simulink model "Resp18e_updatedPulse"  (Simulink 7.3)
settings: Solver=ode23  StartTime=0.0  StopTime=20  FixedStep=0.01  MaxStep=0.05  RelTol=1e-6
values from neighbouring files (symbols this model uses):
  alpha_CO2_brain = 2.9/1e3*760/P_stp/K_stp    (= 0.00097047576489)    [initialize_parameters.m]
  alpha_CO2_fat = 0.9/K_stp/P_stp    (= 0.000396292281489)    [initialize_parameters.m]
  alpha_CO2_heart = 2.4/1e3*760/P_stp/K_stp    (= 0.00080315235715)    [initialize_parameters.m]
  alpha_CO2_lean = 4.2/1e3*760/P_stp/K_stp    (= 0.00140551662501)    [initialize_parameters.m]
  alpha_CO2_lungtiss_fast = alpha_CO2_lungtiss_fast./0.1333    [initialize_parameters.m]
  alpha_CO2_muscle = 4.2/1e3*760/P_stp/K_stp    (= 0.00140551662501)    [initialize_parameters.m]
  alpha_CO2_other = 3.0/1e3*760/P_stp/K_stp    (= 0.00100394044644)    [initialize_parameters.m]
  alpha_O2_fat = 5*0.024/K_stp/P_stp    (= 5.28389708651e-05)    [initialize_parameters.m]
  alpha_O2_tissue = 0.024/K_stp/P_stp    (= 1.0567794173e-05)    [initialize_parameters.m]
  BOHRF0 = O2_SHIFT - T_BLOOD_M_37 * (0.024 + BOHRF * 0.0147) - BOHRF1 * 7.4    (= -3.552)    [initialize_parameters.m]
  BOHRF1 = BOHRF * (1 - T_BLOOD_M_37 * 0.0065)    (= 0.48)    [initialize_parameters.m]
  C_a_CO2_i = 20.8e-3    (= 0.0208)    [initialize_parameters.m]    (also in resp18e_ic_norm.mat = 0.0202734801806)
  C_a_O2_i = 8.95e-3    (= 0.00895)    [initialize_parameters.m]    (also in resp18e_ic_norm.mat = 0.00918087581167)
  CAP_O2 = 0.01 * CAP_O2    (= 0.201)    [initialize_parameters.m]
  Cardiac_duty_cycle = 40    [initialize_parameters.m]
  Co_CO2_brain = 401*K_Co_CO2/1e3/K_stp    (= 0.0107345869894)    [initialize_parameters.m]
  Co_CO2_heart = 487*K_Co_CO2/1e3/K_stp    (= 0.0130367677403)    [initialize_parameters.m]
  Co_CO2_lean = 342*K_Co_CO2/1e3/K_stp    (= 0.00915518391618)    [initialize_parameters.m]
  Co_CO2_muscle = 342*K_Co_CO2/1e3/K_stp    (= 0.00915518391618)    [initialize_parameters.m]
  Co_CO2_other = 355*K_Co_CO2/1e3/K_stp    (= 0.00950318798317)    [initialize_parameters.m]
  DH2ODS = DH2ODS + 0.007 * HB_MEQ * (HB_MEQ - 9) / (13.5 * (13.5 - 9))    (= 0.00498709726946)    [initialize_parameters.m]
  F_insp_alv_alvds = F_v_alv_deadspace / F_insp_hivq    (= 0.00299401197605)    [initialize_parameters.m]
  F_insp_alv_hivq = F_v_alv_hivq      / F_insp_hivq    (= 0.997005988024)    [initialize_parameters.m]
  F_insp_alv_lovq = F_v_alv_lovq      / F_insp_lovq    (= 0.5)    [initialize_parameters.m]
  F_insp_alv_midvq = F_v_alv_midvq     / F_insp_lovq    (= 0.5)    [initialize_parameters.m]
  F_insp_hivq = F_v_alv_deadspace + F_v_alv_hivq    (= 0.334)    [initialize_parameters.m]
  F_insp_lovq = F_v_alv_midvq     + F_v_alv_lovq    (= 0.666)    [initialize_parameters.m]
  Fi_CO2_param_est = 0.01    [initialize_parameters.m]
  Fi_error = 1e-6    (= 1e-06)    [initialize_parameters.m]
  Fi_N2_mean = 1-(Fi_O2_mean + Fi_N2O_mean)    (= 0.65)    [initialize_parameters.m]
  Fi_O2_mean = 0.35    [initialize_parameters.m]
  Fi_O2_param_est = 0.01    [initialize_parameters.m]
  Fq_brain = 0.114    [initialize_parameters.m]
  Fq_error = 1e-8    (= 1e-08)    [initialize_parameters.m]
  Fq_fat = 0.103    [initialize_parameters.m]
  Fq_heart = 0.041    [initialize_parameters.m]
  Fq_hepatic = 0.069    [initialize_parameters.m]
  Fq_kidneys = 0.215    [initialize_parameters.m]
  Fq_lean = 0.090    (= 0.09)    [initialize_parameters.m]
  Fq_lungs_anatomicalshunt = 0.01    [initialize_parameters.m]
  Fq_lungs_hivq = (1-Fq_lungs_pulmshunt-Fq_lungs_anatomicalshunt)    *F_v_alv_hivq/(F_v_alv_hivq+F_v_alv_midvq+F_v_alv_lovq)    (= 0.3)    [initialize_parameters.m]
  Fq_lungs_lovq = (1-Fq_lungs_pulmshunt-Fq_lungs_anatomicalshunt)    *F_v_alv_lovq/(F_v_alv_hivq+F_v_alv_midvq+F_v_alv_lovq)    (= 0.3)    [initialize_parameters.m]
  Fq_lungs_midvq = (1-Fq_lungs_pulmshunt-Fq_lungs_anatomicalshunt)    *F_v_alv_midvq/(F_v_alv_hivq+F_v_alv_midvq+F_v_alv_lovq)    (= 0.3)    [initialize_parameters.m]
  Fq_lungs_pulmshunt = 0.09    [initialize_parameters.m]
  Fq_muscle = 0.096    [initialize_parameters.m]
  Fq_pershunt = 0.101    [initialize_parameters.m]
  Fq_portal = 0.171    [initialize_parameters.m]
  FRC = 2.2    [initialize_parameters.m]
  H2OB = H2OVC + 0.938 * (1 - VC_74)    (= 0.840191964286)    [initialize_parameters.m]
  k_CO2_lungtiss_fast_alvds = k_CO2_lungtiss_fast*F_v_alv_deadspace    (= 3.63090772693e-07)    [initialize_parameters.m]
  k_CO2_lungtiss_fast_hivq = k_CO2_lungtiss_fast*F_v_alv_hivq    (= 0.000120909227307)    [initialize_parameters.m]
  k_CO2_lungtiss_fast_lovq = k_CO2_lungtiss_fast*F_v_alv_lovq    (= 0.000120909227307)    [initialize_parameters.m]
  k_CO2_lungtiss_fast_midvq = k_CO2_lungtiss_fast*F_v_alv_midvq    (= 0.000120909227307)    [initialize_parameters.m]
  k_CO2_lungtiss_slow_alvds = k_CO2_lungtiss_slow*F_v_alv_deadspace    (= 4.95123780945e-09)    [initialize_parameters.m]
  k_CO2_lungtiss_slow_hivq = k_CO2_lungtiss_slow*F_v_alv_hivq    (= 1.64876219055e-06)    [initialize_parameters.m]
  k_CO2_lungtiss_slow_lovq = k_CO2_lungtiss_slow*F_v_alv_lovq    (= 1.64876219055e-06)    [initialize_parameters.m]
  k_CO2_lungtiss_slow_midvq = k_CO2_lungtiss_slow*F_v_alv_midvq    (= 1.64876219055e-06)    [initialize_parameters.m]
  K_diff_CO2_hivq = K_diff_CO2*F_v_alv_hivq    (= 0.0014985)    [initialize_parameters.m]
  K_diff_CO2_lovq = K_diff_CO2*F_v_alv_lovq    (= 0.0014985)    [initialize_parameters.m]
  K_diff_CO2_midvq = K_diff_CO2*F_v_alv_midvq    (= 0.0014985)    [initialize_parameters.m]
  K_diff_O2_hivq = K_diff_O2*F_v_alv_hivq    (= 7.326e-05)    [initialize_parameters.m]
  K_diff_O2_lovq = K_diff_O2*F_v_alv_lovq    (= 7.326e-05)    [initialize_parameters.m]
  K_diff_O2_midvq = K_diff_O2*F_v_alv_midvq    (= 7.326e-05)    [initialize_parameters.m]
  K_exp_alv_alvds = 1/1    (= 1)    [initialize_parameters.m]
  K_exp_alv_hivq = 1/1    (= 1)    [initialize_parameters.m]
  K_press = 760/101.325    (= 7.50061682704)    [initialize_parameters.m]
  K_stp = R*(T_stp+273.15)/(P_stp*1000)    (= 22.4135311621)    [initialize_parameters.m]
  Kg_alv = R*(T_alv+273.15)/(P_baro*1000)    (= 25.3668469802)    [initialize_parameters.m]
  LN10 = 2.30258509299405    (= 2.30258509299)    [initialize_parameters.m]
  m_alv_alvds_i = (FRC-V_deadspace_total)/Kg_alv * F_v_alv_deadspace    [initialize_parameters.m]
  m_alv_hivq_i = (FRC-V_deadspace_total)/Kg_alv * F_v_alv_hivq    [initialize_parameters.m]
  m_alv_lovq_i = (FRC-V_deadspace_total)/Kg_alv * F_v_alv_lovq    [initialize_parameters.m]
  m_alv_midvq_i = (FRC-V_deadspace_total)/Kg_alv * F_v_alv_midvq    [initialize_parameters.m]
  m_CO2_alv_alvds_i = F_CO2_i * m_alv_alvds_i    [initialize_parameters.m]
  m_CO2_alv_hivq_i = F_CO2_i * m_alv_hivq_i    [initialize_parameters.m]
  m_CO2_alv_lovq_i = F_CO2_i * m_alv_lovq_i    [initialize_parameters.m]
  m_CO2_alv_midvq_i = F_CO2_i * m_alv_midvq_i    [initialize_parameters.m]
  m_CO2_brain_b_i = C_a_CO2_i*Vb_brain    (= 0.002184)    [initialize_parameters.m]
  m_CO2_brain_t_i = (Co_CO2_brain  + alpha_CO2_brain *P_v_CO2_i)* Vt_brain    (= 0.0171268217946)    [initialize_parameters.m]
  m_CO2_common_b_i = C_a_CO2_i*Vb_common    (= 0.0170421333333)    [initialize_parameters.m]
  m_CO2_ds0_i = F_CO2_i*m_ds0_i    (= 0.000985538329597)    [initialize_parameters.m]
  m_CO2_ds_large_i = F_CO2_i * m_deadspace_large_1    [initialize_parameters.m]
  m_CO2_ds_med_hivq1_i = F_CO2_i * m_deadspace_med_hivq_1    [initialize_parameters.m]
  m_CO2_ds_med_hivq2_i = F_CO2_i * m_deadspace_med_hivq_2    [initialize_parameters.m]
  m_CO2_ds_med_lovq1_i = F_CO2_i * m_deadspace_med_lovq_1    [initialize_parameters.m]
  m_CO2_ds_med_lovq2_i = F_CO2_i * m_deadspace_med_lovq_2    [initialize_parameters.m]
  m_CO2_ds_small_alvds_i = F_CO2_i * m_deadspace_small_alvdeadspace    [initialize_parameters.m]
  m_CO2_ds_small_hivq_i = F_CO2_i * m_deadspace_small_hivq    [initialize_parameters.m]
  m_CO2_ds_small_lovq_i = F_CO2_i * m_deadspace_small_lovq    [initialize_parameters.m]
  m_CO2_ds_small_midvq_i = F_CO2_i * m_deadspace_small_midvq    [initialize_parameters.m]
  m_CO2_fat_b_i = C_a_CO2_i*Vb_fat    (= 0.0116896)    [initialize_parameters.m]
  m_CO2_fat_t_i = P_a_CO2_i*alpha_CO2_fat*Vt_fat    (= 0.0302752719501)    [initialize_parameters.m]
  m_CO2_heart_b_i = C_a_CO2_i*Vb_heart    (= 0.000832)    [initialize_parameters.m]
  m_CO2_heart_t_i = (Co_CO2_heart  + alpha_CO2_heart *P_v_CO2_i)* Vt_heart    (= 0.00402544335149)    [initialize_parameters.m]
  m_CO2_hepatic_b_i = C_a_CO2_i*Vb_hepatic    (= 0.0019136)    [initialize_parameters.m]
  m_CO2_kidneys_b_i = C_a_CO2_i*Vb_kidneys    (= 0.0012064)    [initialize_parameters.m]
  m_CO2_kidneys_t_i = (Co_CO2_other  + alpha_CO2_other *P_v_CO2_i)* Vt_kidneys    (= 0.0045902552907)    [initialize_parameters.m]
  m_CO2_lean_b_i = C_a_CO2_i*Vb_lean    (= 0.0191984)    [initialize_parameters.m]
  m_CO2_lean_t_i = (Co_CO2_lean   + alpha_CO2_lean  *P_v_CO2_i)* Vt_lean    (= 0.0884995401953)    [initialize_parameters.m]
  m_CO2_liver_t_i = (Co_CO2_other  + alpha_CO2_other *P_v_CO2_i)* Vt_liver    (= 0.0187019339777)    [initialize_parameters.m]
  m_CO2_lungtiss_fast_alvds_i = F_CO2_i*(P_baro-P_A_H2O)*V_lungtiss_alvds *alpha_CO2_lungtiss_fast(2)    [initialize_parameters.m]
  m_CO2_lungtiss_fast_hivq_i = F_CO2_i*(P_baro-P_A_H2O)*V_lungtiss_hivq  *alpha_CO2_lungtiss_fast(2)    [initialize_parameters.m]
  m_CO2_lungtiss_fast_lovq_i = F_CO2_i*(P_baro-P_A_H2O)*V_lungtiss_lovq  *alpha_CO2_lungtiss_fast(2)    [initialize_parameters.m]
  m_CO2_lungtiss_fast_midvq_i = F_CO2_i*(P_baro-P_A_H2O)*V_lungtiss_midvq *alpha_CO2_lungtiss_fast(2)    [initialize_parameters.m]
  m_CO2_lungtiss_slow_alvds_i = F_CO2_i*(P_baro-P_A_H2O)*V_lungtiss_alvds*alpha_CO2_lungtiss_slow    [initialize_parameters.m]
  m_CO2_lungtiss_slow_hivq_i = F_CO2_i*(P_baro-P_A_H2O)*V_lungtiss_hivq *alpha_CO2_lungtiss_slow    [initialize_parameters.m]
  m_CO2_lungtiss_slow_lovq_i = F_CO2_i*(P_baro-P_A_H2O)*V_lungtiss_lovq *alpha_CO2_lungtiss_slow    [initialize_parameters.m]
  m_CO2_lungtiss_slow_midvq_i = F_CO2_i*(P_baro-P_A_H2O)*V_lungtiss_midvq*alpha_CO2_lungtiss_slow    [initialize_parameters.m]
  m_CO2_LV_b_i = C_a_CO2_i*Vb_LV    (= 0.00391733333333)    [initialize_parameters.m]
  m_CO2_muscle_b_i = C_a_CO2_i*Vb_muscle    (= 0.0201344)    [initialize_parameters.m]
  m_CO2_muscle_t_i = (Co_CO2_muscle + alpha_CO2_muscle*P_v_CO2_i)* Vt_muscle    (= 0.363660431061)    [initialize_parameters.m]
  m_CO2_pershunt_b_i = C_a_CO2_i*Vb_pershunt    (= 0.0027248)    [initialize_parameters.m]
  m_CO2_portal_b_i = C_a_CO2_i*Vb_portal    (= 0.0210912)    [initialize_parameters.m]
  m_CO2_portal_t_i = (Co_CO2_other  + alpha_CO2_other *P_v_CO2_i)* Vt_portal    (= 0.0164739329706)    [initialize_parameters.m]
  m_CO2_pulmcap_b_hivq_i = C_a_CO2_i*Vb_pulmcap_hivq    (= 0.000630933333333)    [initialize_parameters.m]
  m_CO2_pulmcap_b_lovq_i = C_a_CO2_i*Vb_pulmcap_lovq    (= 0.000630933333333)    [initialize_parameters.m]
  m_CO2_pulmcap_b_midvq_i = C_a_CO2_i*Vb_pulmcap_midvq    (= 0.000630933333333)    [initialize_parameters.m]
  m_CO2_pulmcap_b_pulmshunt_i = C_a_CO2_i*Vb_pulmcap_pulmshunt    (= 0.0001872)    [initialize_parameters.m]
  m_CO2_RV_b_i = C_v_CO2_i*Vb_RV    (= 0.004181)    [initialize_parameters.m]
  m_N2_alv_alvds_i = Fi_N2_mean * (m_alv_alvds_i - m_CO2_alv_alvds_i)    [initialize_parameters.m]
  ... (+122 more)
undefined symbols (not defined in the file or in its folder): AH2OVC, AHCO3B, DHCO3BDS, litres, mole
libraries: simulink x28
(part 3 of 8)

== system Resp18e_updatedPulse/Patient/Airways + alveoli/Series dead Space alv dead sp ==
  Insp flow in : Inport  PortDimensions=4  OutDataType=sfix(16)  OutScaling=2^0
  Exp flow in : Inport  Port=2  PortDimensions=4  OutDataType=sfix(16)  OutScaling=2^0
  1/u : Math  Operator=reciprocal  OutDataType=sfix(16)  OutScaling=2^0  SaturateOnIntegerOverflow=on
  CO2 : Integrator  InitialCondition=m_CO2_ds_small_alvds_i
  N2 : Integrator  InitialCondition=m_N2_ds_small_alvds_i
  N2O : Integrator  InitialCondition=m_N2O_ds_small_alvds_i
  N2O O2 CO2 N2 : Demux
  "N2O O2 CO2 N2 " : Demux
  N2O,O2 CO2,N22 : Mux
  N2O,O2 CO2,N23 : Mux
  O2 : Integrator  InitialCondition=m_O2_ds_small_alvds_i
  P{2..13} (12 alike) : Product  OutDataType=sfix(16)  OutScaling=2^0  SaturateOnIntegerOverflow=on  RndMeth=Zero  InputSameDT=on  OutDataTypeStr=Inherit: Same as first input
  Vds gas vol : Sum  Inputs=++++  OutDataType=sfix(16)  OutScaling=2^0  SaturateOnIntegerOverflow=on  InputSameDT=on  OutDataTypeStr=Inherit: Same as first input
  sum : Sum  Inputs=--++  OutDataType=sfix(16)  OutScaling=2^0  SaturateOnIntegerOverflow=on  InputSameDT=on  OutDataTypeStr=Inherit: Same as first input
  sum1 : Sum  Inputs=+-+-  OutDataType=sfix(16)  OutScaling=2^0  SaturateOnIntegerOverflow=on  InputSameDT=on  OutDataTypeStr=Inherit: Same as first input
  sum2 : Sum  Inputs=-++-  OutDataType=sfix(16)  OutScaling=2^0  SaturateOnIntegerOverflow=on  InputSameDT=on  OutDataTypeStr=Inherit: Same as first input
  sum3 : Sum  Inputs=-++-  OutDataType=sfix(16)  OutScaling=2^0  SaturateOnIntegerOverflow=on  InputSameDT=on  OutDataTypeStr=Inherit: Same as first input
  sum4 : Sum  Inputs=++++  OutDataType=sfix(16)  OutScaling=2^0  SaturateOnIntegerOverflow=on  InputSameDT=on  OutDataTypeStr=Inherit: Same as first input
  sum5 : Sum  Inputs=++++  OutDataType=sfix(16)  OutScaling=2^0  SaturateOnIntegerOverflow=on  InputSameDT=on  OutDataTypeStr=Inherit: Same as first input
  Insp flow  Out: : Outport  OutDataType=sfix(16)  OutScaling=2^0
  Exp flow  Out: : Outport  Port=2  OutDataType=sfix(16)  OutScaling=2^0
  wires:
  Insp flow in/1 -> "N2O O2 CO2 N2 "/1
  "N2O O2 CO2 N2 "/4 -> sum4/4, sum3/3
  "N2O O2 CO2 N2 "/3 -> sum4/3, sum2/3
  "N2O O2 CO2 N2 "/2 -> sum4/2, sum1/3
  "N2O O2 CO2 N2 "/1 -> sum4/1, sum/4
  Exp flow in/1 -> N2O O2 CO2 N2/1
  N2O O2 CO2 N2/4 -> sum5/4, sum3/2
  N2O O2 CO2 N2/3 -> sum5/3, sum2/2
  N2O O2 CO2 N2/2 -> sum5/2, sum1/1
  N2O O2 CO2 N2/1 -> sum5/1, sum/3
  sum5/1 -> P6/2, P5/2, P10/2, P11/1
  sum4/1 -> P13/1, P9/1, P7/1, P4/1
  N2/1 -> Vds gas vol/4, P12/2
  P5/1 -> sum/1, N2O,O2 CO2,N23/1
  P6/1 -> sum1/4, N2O,O2 CO2,N23/2
  O2/1 -> Vds gas vol/2, P3/2
  N2O/1 -> Vds gas vol/1, P2/1
  P7/1 -> sum1/2, N2O,O2 CO2,N22/2
  1/u/1 -> P2/2, P3/1, P8/1, P12/1
  Vds gas vol/1 -> 1/u/1
  sum1/1 -> O2/1
  sum/1 -> N2O/1
  sum2/1 -> CO2/1
  P2/1 -> P5/1, P4/2
  CO2/1 -> P8/2, Vds gas vol/3
  P8/1 -> P10/1, P9/2
  P10/1 -> sum2/4, N2O,O2 CO2,N23/3
  N2O,O2 CO2,N23/1 -> Exp flow  Out:/1
  N2O,O2 CO2,N22/1 -> Insp flow  Out:/1
  P4/1 -> N2O,O2 CO2,N22/1, sum/2
  P9/1 -> N2O,O2 CO2,N22/3, sum2/1
  sum3/1 -> N2/1
  P12/1 -> P11/2, P13/2
  P13/1 -> sum3/1, N2O,O2 CO2,N22/4
  P3/1 -> P6/1, P7/2
  P11/1 -> sum3/4, N2O,O2 CO2,N23/4

== system Resp18e_updatedPulse/Patient/Airways + alveoli/Series dead Space hi V/Q ==
  Insp flow in : Inport  PortDimensions=4  OutDataType=sfix(16)  OutScaling=2^0
  Exp flow in : Inport  Port=2  PortDimensions=4  OutDataType=sfix(16)  OutScaling=2^0
  1/u : Math  Operator=reciprocal  OutDataType=sfix(16)  OutScaling=2^0  SaturateOnIntegerOverflow=on
  CO2 : Integrator  InitialCondition=m_CO2_ds_small_hivq_i
  N2 : Integrator  InitialCondition=m_N2_ds_small_hivq_i
  N2O : Integrator  InitialCondition=m_N2O_ds_small_hivq_i
  N2O O2 CO2 N2 : Demux
  "N2O O2 CO2 N2 " : Demux
  N2O,O2 CO2,N22 : Mux
  N2O,O2 CO2,N23 : Mux
  O2 : Integrator  InitialCondition=m_O2_ds_small_hivq_i
  P{2..13} (12 alike) : Product  OutDataType=sfix(16)  OutScaling=2^0  SaturateOnIntegerOverflow=on  RndMeth=Zero  InputSameDT=on  OutDataTypeStr=Inherit: Same as first input
  Vds gas vol : Sum  Inputs=++++  OutDataType=sfix(16)  OutScaling=2^0  SaturateOnIntegerOverflow=on  InputSameDT=on  OutDataTypeStr=Inherit: Same as first input
  sum : Sum  Inputs=--++  OutDataType=sfix(16)  OutScaling=2^0  SaturateOnIntegerOverflow=on  InputSameDT=on  OutDataTypeStr=Inherit: Same as first input
  sum1 : Sum  Inputs=+-+-  OutDataType=sfix(16)  OutScaling=2^0  SaturateOnIntegerOverflow=on  InputSameDT=on  OutDataTypeStr=Inherit: Same as first input
  sum2 : Sum  Inputs=-++-  OutDataType=sfix(16)  OutScaling=2^0  SaturateOnIntegerOverflow=on  InputSameDT=on  OutDataTypeStr=Inherit: Same as first input
  sum3 : Sum  Inputs=-++-  OutDataType=sfix(16)  OutScaling=2^0  SaturateOnIntegerOverflow=on  InputSameDT=on  OutDataTypeStr=Inherit: Same as first input
  sum4 : Sum  Inputs=++++  OutDataType=sfix(16)  OutScaling=2^0  SaturateOnIntegerOverflow=on  InputSameDT=on  OutDataTypeStr=Inherit: Same as first input
  sum5 : Sum  Inputs=++++  OutDataType=sfix(16)  OutScaling=2^0  SaturateOnIntegerOverflow=on  InputSameDT=on  OutDataTypeStr=Inherit: Same as first input
  Insp flow  Out: : Outport  OutDataType=sfix(16)  OutScaling=2^0
  Exp flow  Out: : Outport  Port=2  OutDataType=sfix(16)  OutScaling=2^0
  wires:
  P11/1 -> N2O,O2 CO2,N23/4, sum3/4
  P3/1 -> P7/2, P6/1
  P13/1 -> N2O,O2 CO2,N22/4, sum3/1
  P12/1 -> P13/2, P11/2
  sum3/1 -> N2/1
  P9/1 -> sum2/1, N2O,O2 CO2,N22/3
  P4/1 -> sum/2, N2O,O2 CO2,N22/1
  N2O,O2 CO2,N22/1 -> Insp flow  Out:/1
  N2O,O2 CO2,N23/1 -> Exp flow  Out:/1
  P10/1 -> N2O,O2 CO2,N23/3, sum2/4
  P8/1 -> P9/2, P10/1
  CO2/1 -> Vds gas vol/3, P8/2
  P2/1 -> P4/2, P5/1
  sum2/1 -> CO2/1
  sum/1 -> N2O/1
  sum1/1 -> O2/1
  Vds gas vol/1 -> 1/u/1
  1/u/1 -> P12/1, P8/1, P3/1, P2/2
  P7/1 -> N2O,O2 CO2,N22/2, sum1/2
  N2O/1 -> P2/1, Vds gas vol/1
  O2/1 -> P3/2, Vds gas vol/2
  P6/1 -> N2O,O2 CO2,N23/2, sum1/4
  P5/1 -> N2O,O2 CO2,N23/1, sum/1
  N2/1 -> P12/2, Vds gas vol/4
  sum4/1 -> P4/1, P7/1, P9/1, P13/1
  sum5/1 -> P11/1, P10/2, P5/2, P6/2
  N2O O2 CO2 N2/1 -> sum/3, sum5/1
  N2O O2 CO2 N2/2 -> sum1/1, sum5/2
  N2O O2 CO2 N2/3 -> sum2/2, sum5/3
  N2O O2 CO2 N2/4 -> sum3/2, sum5/4
  Exp flow in/1 -> N2O O2 CO2 N2/1
  "N2O O2 CO2 N2 "/1 -> sum/4, sum4/1
  "N2O O2 CO2 N2 "/2 -> sum1/3, sum4/2
  "N2O O2 CO2 N2 "/3 -> sum2/3, sum4/3
  "N2O O2 CO2 N2 "/4 -> sum3/3, sum4/4
  Insp flow in/1 -> "N2O O2 CO2 N2 "/1

== system Resp18e_updatedPulse/Patient/Airways + alveoli/Series dead Space lo V/Q ==
  Insp flow in : Inport  PortDimensions=4  OutDataType=sfix(16)  OutScaling=2^0
  Exp flow in : Inport  Port=2  PortDimensions=4  OutDataType=sfix(16)  OutScaling=2^0
  1/u : Math  Operator=reciprocal  OutDataType=sfix(16)  OutScaling=2^0  SaturateOnIntegerOverflow=on
  CO2 : Integrator  InitialCondition=m_CO2_ds_small_lovq_i
  N2 : Integrator  InitialCondition=m_N2_ds_small_lovq_i
  N2O : Integrator  InitialCondition=m_N2O_ds_small_lovq_i
  N2O O2 CO2 N2 : Demux
  "N2O O2 CO2 N2 " : Demux
  N2O,O2 CO2,N22 : Mux
  N2O,O2 CO2,N23 : Mux
  O2 : Integrator  InitialCondition=m_O2_ds_small_lovq_i
  P{2..13} (12 alike) : Product  OutDataType=sfix(16)  OutScaling=2^0  SaturateOnIntegerOverflow=on  RndMeth=Zero  InputSameDT=on  OutDataTypeStr=Inherit: Same as first input
  Vds gas vol : Sum  Inputs=++++  OutDataType=sfix(16)  OutScaling=2^0  SaturateOnIntegerOverflow=on  InputSameDT=on  OutDataTypeStr=Inherit: Same as first input
  sum : Sum  Inputs=--++  OutDataType=sfix(16)  OutScaling=2^0  SaturateOnIntegerOverflow=on  InputSameDT=on  OutDataTypeStr=Inherit: Same as first input
  sum1 : Sum  Inputs=+-+-  OutDataType=sfix(16)  OutScaling=2^0  SaturateOnIntegerOverflow=on  InputSameDT=on  OutDataTypeStr=Inherit: Same as first input
  sum2 : Sum  Inputs=-++-  OutDataType=sfix(16)  OutScaling=2^0  SaturateOnIntegerOverflow=on  InputSameDT=on  OutDataTypeStr=Inherit: Same as first input
  sum3 : Sum  Inputs=-++-  OutDataType=sfix(16)  OutScaling=2^0  SaturateOnIntegerOverflow=on  InputSameDT=on  OutDataTypeStr=Inherit: Same as first input
  sum4 : Sum  Inputs=++++  OutDataType=sfix(16)  OutScaling=2^0  SaturateOnIntegerOverflow=on  InputSameDT=on  OutDataTypeStr=Inherit: Same as first input
  sum5 : Sum  Inputs=++++  OutDataType=sfix(16)  OutScaling=2^0  SaturateOnIntegerOverflow=on  InputSameDT=on  OutDataTypeStr=Inherit: Same as first input
  Insp flow  Out: : Outport  OutDataType=sfix(16)  OutScaling=2^0
  Exp flow  Out: : Outport  Port=2  OutDataType=sfix(16)  OutScaling=2^0
  wires:
  P11/1 -> N2O,O2 CO2,N23/4, sum3/4
  P3/1 -> P7/2, P6/1
  P13/1 -> N2O,O2 CO2,N22/4, sum3/1
  P12/1 -> P13/2, P11/2
  sum3/1 -> N2/1
  P9/1 -> sum2/1, N2O,O2 CO2,N22/3
  P4/1 -> sum/2, N2O,O2 CO2,N22/1
  N2O,O2 CO2,N22/1 -> Insp flow  Out:/1
  N2O,O2 CO2,N23/1 -> Exp flow  Out:/1
  P10/1 -> N2O,O2 CO2,N23/3, sum2/4
  P8/1 -> P9/2, P10/1
  CO2/1 -> Vds gas vol/3, P8/2
  P2/1 -> P4/2, P5/1
  sum2/1 -> CO2/1
  sum/1 -> N2O/1
  sum1/1 -> O2/1
  Vds gas vol/1 -> 1/u/1
  1/u/1 -> P12/1, P8/1, P3/1, P2/2
  P7/1 -> N2O,O2 CO2,N22/2, sum1/2
  N2O/1 -> P2/1, Vds gas vol/1
  O2/1 -> P3/2, Vds gas vol/2
  P6/1 -> N2O,O2 CO2,N23/2, sum1/4
  P5/1 -> N2O,O2 CO2,N23/1, sum/1
  N2/1 -> P12/2, Vds gas vol/4
  sum4/1 -> P4/1, P7/1, P9/1, P13/1
  sum5/1 -> P11/1, P10/2, P5/2, P6/2
  N2O O2 CO2 N2/1 -> sum/3, sum5/1
  N2O O2 CO2 N2/2 -> sum1/1, sum5/2
  N2O O2 CO2 N2/3 -> sum2/2, sum5/3
  N2O O2 CO2 N2/4 -> sum3/2, sum5/4
  Exp flow in/1 -> N2O O2 CO2 N2/1
  "N2O O2 CO2 N2 "/1 -> sum/4, sum4/1
  "N2O O2 CO2 N2 "/2 -> sum1/3, sum4/2
  "N2O O2 CO2 N2 "/3 -> sum2/3, sum4/3
  "N2O O2 CO2 N2 "/4 -> sum3/3, sum4/4
  Insp flow in/1 -> "N2O O2 CO2 N2 "/1

== system Resp18e_updatedPulse/Patient/Airways + alveoli/Series dead Space mid V/Q ==
  Insp flow in : Inport  PortDimensions=4  OutDataType=sfix(16)  OutScaling=2^0
  Exp flow in : Inport  Port=2  PortDimensions=4  OutDataType=sfix(16)  OutScaling=2^0
  1/u : Math  Operator=reciprocal  OutDataType=sfix(16)  OutScaling=2^0  SaturateOnIntegerOverflow=on
  CO2 : Integrator  InitialCondition=m_CO2_ds_small_midvq_i
  N2 : Integrator  InitialCondition=m_N2_ds_small_midvq_i
  N2O : Integrator  InitialCondition=m_N2O_ds_small_midvq_i
  N2O O2 CO2 N2 : Demux
  "N2O O2 CO2 N2 " : Demux
  N2O,O2 CO2,N22 : Mux
  N2O,O2 CO2,N23 : Mux
  O2 : Integrator  InitialCondition=m_O2_ds_small_midvq_i
  P{2..13} (12 alike) : Product  OutDataType=sfix(16)  OutScaling=2^0  SaturateOnIntegerOverflow=on  RndMeth=Zero  InputSameDT=on  OutDataTypeStr=Inherit: Same as first input
  Sum Exp flow : Sum  Inputs=++++  OutDataType=sfix(16)  OutScaling=2^0  SaturateOnIntegerOverflow=on  InputSameDT=on  OutDataTypeStr=Inherit: Same as first input
  Sum Insp flow : Sum  Inputs=++++  OutDataType=sfix(16)  OutScaling=2^0  SaturateOnIntegerOverflow=on  InputSameDT=on  OutDataTypeStr=Inherit: Same as first input
  Vds gas vol : Sum  Inputs=++++  OutDataType=sfix(16)  OutScaling=2^0  SaturateOnIntegerOverflow=on  InputSameDT=on  OutDataTypeStr=Inherit: Same as first input
  sum : Sum  Inputs=--++  OutDataType=sfix(16)  OutScaling=2^0  SaturateOnIntegerOverflow=on  InputSameDT=on  OutDataTypeStr=Inherit: Same as first input
  sum1 : Sum  Inputs=+-+-  OutDataType=sfix(16)  OutScaling=2^0  SaturateOnIntegerOverflow=on  InputSameDT=on  OutDataTypeStr=Inherit: Same as first input
  sum2 : Sum  Inputs=-++-  OutDataType=sfix(16)  OutScaling=2^0  SaturateOnIntegerOverflow=on  InputSameDT=on  OutDataTypeStr=Inherit: Same as first input
  sum3 : Sum  Inputs=-++-  OutDataType=sfix(16)  OutScaling=2^0  SaturateOnIntegerOverflow=on  InputSameDT=on  OutDataTypeStr=Inherit: Same as first input
  Insp flow  Out: : Outport  OutDataType=sfix(16)  OutScaling=2^0
  Exp flow  Out: : Outport  Port=2  OutDataType=sfix(16)  OutScaling=2^0
  wires:
  Insp flow in/1 -> "N2O O2 CO2 N2 "/1
  "N2O O2 CO2 N2 "/4 -> Sum Insp flow/4, sum3/3
  "N2O O2 CO2 N2 "/3 -> Sum Insp flow/3, sum2/3
  "N2O O2 CO2 N2 "/2 -> Sum Insp flow/2, sum1/3
  "N2O O2 CO2 N2 "/1 -> Sum Insp flow/1, sum/4
  Exp flow in/1 -> N2O O2 CO2 N2/1
  N2O O2 CO2 N2/4 -> Sum Exp flow/4, sum3/2
  N2O O2 CO2 N2/3 -> Sum Exp flow/3, sum2/2
  N2O O2 CO2 N2/2 -> Sum Exp flow/2, sum1/1
  N2O O2 CO2 N2/1 -> Sum Exp flow/1, sum/3
  Sum Exp flow/1 -> P6/2, P5/2, P10/2, P11/1
  Sum Insp flow/1 -> P13/1, P9/1, P7/1, P4/1
  N2/1 -> Vds gas vol/4, P12/2
  P5/1 -> sum/1, N2O,O2 CO2,N23/1
  P6/1 -> sum1/4, N2O,O2 CO2,N23/2
  O2/1 -> Vds gas vol/2, P3/2
  N2O/1 -> Vds gas vol/1, P2/1
  P7/1 -> sum1/2, N2O,O2 CO2,N22/2
  1/u/1 -> P2/2, P3/1, P8/1, P12/1
  Vds gas vol/1 -> 1/u/1
  sum1/1 -> O2/1
  sum/1 -> N2O/1
  sum2/1 -> CO2/1
  P2/1 -> P5/1, P4/2
  CO2/1 -> P8/2, Vds gas vol/3
  P8/1 -> P10/1, P9/2
  P10/1 -> sum2/4, N2O,O2 CO2,N23/3
  N2O,O2 CO2,N23/1 -> Exp flow  Out:/1
  N2O,O2 CO2,N22/1 -> Insp flow  Out:/1
  P4/1 -> N2O,O2 CO2,N22/1, sum/2
  P9/1 -> N2O,O2 CO2,N22/3, sum2/1
  sum3/1 -> N2/1
  P12/1 -> P11/2, P13/2
  P13/1 -> sum3/1, N2O,O2 CO2,N22/4
  P3/1 -> P6/1, P7/2
  P11/1 -> sum3/4, N2O,O2 CO2,N23/4

== system Resp18e_updatedPulse/Patient/Airways + alveoli/Series deadspace large_1 ==
  mdot insp total : Inport  PortDimensions=1  OutDataType=sfix(16)  OutScaling=2^0
  Insp flow in : Inport  Port=2  PortDimensions=4  OutDataType=sfix(16)  OutScaling=2^0
  mdot exp Total : Inport  Port=3  PortDimensions=1  OutDataType=sfix(16)  OutScaling=2^0
  Exp flow in : Inport  Port=4  PortDimensions=4  OutDataType=sfix(16)  OutScaling=2^0
  1/u : Math  Operator=reciprocal  OutDataType=sfix(16)  OutScaling=2^0  SaturateOnIntegerOverflow=on
  CO2 : Integrator  InitialCondition=m_CO2_ds_large_i
  N2 : Integrator  InitialCondition=m_N2_ds_large_i
  N2O : Integrator  InitialCondition=m_N2O_ds_large_i
  N2O,O2 CO2,N2 : Demux
  N2O,O2 CO2,N21 : Demux
  N2O,O2 CO2,N22 : Mux
  N2O,O2 CO2,N23 : Mux
  O2 : Integrator  InitialCondition=m_O2_ds_large_i
  P{2..13} (12 alike) : Product  OutDataType=sfix(16)  OutScaling=2^0  SaturateOnIntegerOverflow=on  RndMeth=Zero  InputSameDT=on  OutDataTypeStr=Inherit: Same as first input
  To WS3 : ToWorkspace  VariableName=m_large1_ds  SampleTime=t_sample  SaveFormat=Array
  Vds gas vol : Sum  Inputs=++++  OutDataType=sfix(16)  OutScaling=2^0  SaturateOnIntegerOverflow=on  InputSameDT=on  OutDataTypeStr=Inherit: Same as first input
  sum : Sum  Inputs=--++  OutDataType=sfix(16)  OutScaling=2^0  SaturateOnIntegerOverflow=on  InputSameDT=on  OutDataTypeStr=Inherit: Same as first input
  sum1 : Sum  Inputs=+-+-  OutDataType=sfix(16)  OutScaling=2^0  SaturateOnIntegerOverflow=on  InputSameDT=on  OutDataTypeStr=Inherit: Same as first input
  sum2 : Sum  Inputs=-++-  OutDataType=sfix(16)  OutScaling=2^0  SaturateOnIntegerOverflow=on  InputSameDT=on  OutDataTypeStr=Inherit: Same as first input
  sum3 : Sum  Inputs=-++-  OutDataType=sfix(16)  OutScaling=2^0  SaturateOnIntegerOverflow=on  InputSameDT=on  OutDataTypeStr=Inherit: Same as first input
  Insp flow  Out: : Outport  OutDataType=sfix(16)  OutScaling=2^0
  Exp flow  Out: : Outport  Port=2  OutDataType=sfix(16)  OutScaling=2^0
  wires:
  N2/1 -> Vds gas vol/4, P12/2
  P12/1 -> P11/2, P13/2
  P5/1 -> sum/1, N2O,O2 CO2,N23/1
  P6/1 -> sum1/4, N2O,O2 CO2,N23/2
  O2/1 -> Vds gas vol/2, P3/2
  N2O/1 -> Vds gas vol/1, P2/1
  P7/1 -> sum1/2, N2O,O2 CO2,N22/2
  1/u/1 -> P2/2, P3/1, P8/1, P12/1
  sum1/1 -> O2/1
  sum/1 -> N2O/1
  mdot insp total/1 -> P4/1, P9/1, P13/1, P7/1
  sum2/1 -> CO2/1
  P2/1 -> P5/1, P4/2
  CO2/1 -> P8/2, Vds gas vol/3
  P8/1 -> P10/1, P9/2
  mdot exp Total/1 -> P6/2, P5/2, P10/2, P11/1
  P10/1 -> sum2/4, N2O,O2 CO2,N23/3
  N2O,O2 CO2,N23/1 -> Exp flow  Out:/1
  N2O,O2 CO2,N22/1 -> Insp flow  Out:/1
  Exp flow in/1 -> N2O,O2 CO2,N2/1
  N2O,O2 CO2,N2/2 -> sum1/1
  Insp flow in/1 -> N2O,O2 CO2,N21/1
  N2O,O2 CO2,N21/1 -> sum/4
  N2O,O2 CO2,N21/2 -> sum1/3
  N2O,O2 CO2,N21/3 -> sum2/3
  P4/1 -> N2O,O2 CO2,N22/1, sum/2
  N2O,O2 CO2,N2/1 -> sum/3
  P9/1 -> N2O,O2 CO2,N22/3, sum2/1
  N2O,O2 CO2,N2/3 -> sum2/2
  sum3/1 -> N2/1
  N2O,O2 CO2,N2/4 -> sum3/2
  N2O,O2 CO2,N21/4 -> sum3/3
  P13/1 -> sum3/1, N2O,O2 CO2,N22/4
  P3/1 -> P6/1, P7/2
  P11/1 -> sum3/4, N2O,O2 CO2,N23/4
  Vds gas vol/1 -> 1/u/1, To WS3/1

== system Resp18e_updatedPulse/Patient/Airways + alveoli/Series deadspace large_2 ==
  mdot insp total : Inport  PortDimensions=1  OutDataType=sfix(16)  OutScaling=2^0
  Insp flow in : Inport  Port=2  PortDimensions=4  OutDataType=sfix(16)  OutScaling=2^0
  mdot exp total : Inport  Port=3  PortDimensions=1  OutDataType=sfix(16)  OutScaling=2^0
  Exp flow in : Inport  Port=4  PortDimensions=4  OutDataType=sfix(16)  OutScaling=2^0
  1/u : Math  Operator=reciprocal  OutDataType=sfix(16)  OutScaling=2^0  SaturateOnIntegerOverflow=on
  CO2 : Integrator  InitialCondition=m_CO2_ds_large_i
  N2 : Integrator  InitialCondition=m_N2_ds_large_i
  N2O : Integrator  InitialCondition=m_N2O_ds_large_i
  N2O,O2 CO2,N2 : Demux
  N2O,O2 CO2,N21 : Demux
  N2O,O2 CO2,N22 : Mux
  N2O,O2 CO2,N23 : Mux
  O2 : Integrator  InitialCondition=m_O2_ds_large_i
  P{2..13} (12 alike) : Product  OutDataType=sfix(16)  OutScaling=2^0  SaturateOnIntegerOverflow=on  RndMeth=Zero  InputSameDT=on  OutDataTypeStr=Inherit: Same as first input
  Vds gas vol : Sum  Inputs=++++  OutDataType=sfix(16)  OutScaling=2^0  SaturateOnIntegerOverflow=on  InputSameDT=on  OutDataTypeStr=Inherit: Same as first input
  sum : Sum  Inputs=--++  OutDataType=sfix(16)  OutScaling=2^0  SaturateOnIntegerOverflow=on  InputSameDT=on  OutDataTypeStr=Inherit: Same as first input
  sum1 : Sum  Inputs=+-+-  OutDataType=sfix(16)  OutScaling=2^0  SaturateOnIntegerOverflow=on  InputSameDT=on  OutDataTypeStr=Inherit: Same as first input
  sum2 : Sum  Inputs=-++-  OutDataType=sfix(16)  OutScaling=2^0  SaturateOnIntegerOverflow=on  InputSameDT=on  OutDataTypeStr=Inherit: Same as first input
  sum3 : Sum  Inputs=-++-  OutDataType=sfix(16)  OutScaling=2^0  SaturateOnIntegerOverflow=on  InputSameDT=on  OutDataTypeStr=Inherit: Same as first input
  Insp flow  Out: : Outport  OutDataType=sfix(16)  OutScaling=2^0
  Exp flow  Out: : Outport  Port=2  OutDataType=sfix(16)  OutScaling=2^0
  wires:
  N2/1 -> Vds gas vol/4, P12/2
  P11/1 -> N2O,O2 CO2,N23/4, sum3/4
  P3/1 -> P6/1, P7/2
  P13/1 -> N2O,O2 CO2,N22/4, sum3/1
  N2O,O2 CO2,N21/4 -> sum3/3
  N2O,O2 CO2,N2/4 -> sum3/2
  P12/1 -> P11/2, P13/2
  sum3/1 -> N2/1
  N2O,O2 CO2,N2/3 -> sum2/2
  P9/1 -> sum2/1, N2O,O2 CO2,N22/3
  N2O,O2 CO2,N2/1 -> sum/3
  P4/1 -> sum/2, N2O,O2 CO2,N22/1
  N2O,O2 CO2,N21/3 -> sum2/3
  N2O,O2 CO2,N21/2 -> sum1/3
  N2O,O2 CO2,N21/1 -> sum/4
  Insp flow in/1 -> N2O,O2 CO2,N21/1
  N2O,O2 CO2,N2/2 -> sum1/1
  Exp flow in/1 -> N2O,O2 CO2,N2/1
  N2O,O2 CO2,N22/1 -> Insp flow  Out:/1
  N2O,O2 CO2,N23/1 -> Exp flow  Out:/1
  P10/1 -> N2O,O2 CO2,N23/3, sum2/4
  mdot exp total/1 -> P11/1, P10/2, P5/2, P6/2
  P8/1 -> P10/1, P9/2
  CO2/1 -> P8/2, Vds gas vol/3
  P2/1 -> P5/1, P4/2
  sum2/1 -> CO2/1
  mdot insp total/1 -> P7/1, P13/1, P9/1, P4/1
  sum/1 -> N2O/1
  sum1/1 -> O2/1
  Vds gas vol/1 -> 1/u/1
  1/u/1 -> P12/1, P8/1, P3/1, P2/2
  P7/1 -> N2O,O2 CO2,N22/2, sum1/2
  N2O/1 -> P2/1, Vds gas vol/1
  O2/1 -> P3/2, Vds gas vol/2
  P6/1 -> N2O,O2 CO2,N23/2, sum1/4
  P5/1 -> N2O,O2 CO2,N23/1, sum/1

== system Resp18e_updatedPulse/Patient/Airways + alveoli/Series deadspace large_3 ==
  mdot insp total : Inport  PortDimensions=1  OutDataType=sfix(16)  OutScaling=2^0
  Insp flow in : Inport  Port=2  PortDimensions=4  OutDataType=sfix(16)  OutScaling=2^0
  Exp flow in : Inport  Port=3  PortDimensions=4  OutDataType=sfix(16)  OutScaling=2^0
  1/u : Math  Operator=reciprocal  OutDataType=sfix(16)  OutScaling=2^0  SaturateOnIntegerOverflow=on
  CO2 : Integrator  InitialCondition=m_CO2_ds_large_i
  N2 : Integrator  InitialCondition=m_N2_ds_large_i
  N2O : Integrator  InitialCondition=m_N2O_ds_large_i
  N2O,O2 CO2,N2 : Demux
  N2O,O2 CO2,N21 : Demux
  N2O,O2 CO2,N22 : Mux
  N2O,O2 CO2,N23 : Mux
  O2 : Integrator  InitialCondition=m_O2_ds_large_i
  P{2..13} (12 alike) : Product  OutDataType=sfix(16)  OutScaling=2^0  SaturateOnIntegerOverflow=on  RndMeth=Zero  InputSameDT=on  OutDataTypeStr=Inherit: Same as first input
  Vds gas vol : Sum  Inputs=++++  OutDataType=sfix(16)  OutScaling=2^0  SaturateOnIntegerOverflow=on  InputSameDT=on  OutDataTypeStr=Inherit: Same as first input
  mdot_exp : Sum  Inputs=++++  OutDataType=sfix(16)  OutScaling=2^0  SaturateOnIntegerOverflow=on  InputSameDT=on  OutDataTypeStr=Inherit: Same as first input
  sum : Sum  Inputs=--++  OutDataType=sfix(16)  OutScaling=2^0  SaturateOnIntegerOverflow=on  InputSameDT=on  OutDataTypeStr=Inherit: Same as first input
  sum1 : Sum  Inputs=+-+-  OutDataType=sfix(16)  OutScaling=2^0  SaturateOnIntegerOverflow=on  InputSameDT=on  OutDataTypeStr=Inherit: Same as first input
  sum2 : Sum  Inputs=-++-  OutDataType=sfix(16)  OutScaling=2^0  SaturateOnIntegerOverflow=on  InputSameDT=on  OutDataTypeStr=Inherit: Same as first input
  sum3 : Sum  Inputs=-++-  OutDataType=sfix(16)  OutScaling=2^0  SaturateOnIntegerOverflow=on  InputSameDT=on  OutDataTypeStr=Inherit: Same as first input
  Insp flow  Out: : Outport  OutDataType=sfix(16)  OutScaling=2^0
  Exp flow  Out: : Outport  Port=2  OutDataType=sfix(16)  OutScaling=2^0
  mdot exp total : Outport  Port=3  OutDataType=sfix(16)  OutScaling=2^0
  wires:
  P5/1 -> sum/1, N2O,O2 CO2,N23/1
  P6/1 -> sum1/4, N2O,O2 CO2,N23/2
  O2/1 -> Vds gas vol/2, P3/2
  N2O/1 -> Vds gas vol/1, P2/1
  P7/1 -> sum1/2, N2O,O2 CO2,N22/2
  1/u/1 -> P2/2, P3/1, P8/1, P12/1
  Vds gas vol/1 -> 1/u/1
  sum1/1 -> O2/1
  sum/1 -> N2O/1
  mdot insp total/1 -> P4/1, P9/1, P13/1, P7/1
  sum2/1 -> CO2/1
  P2/1 -> P4/2, P5/1
  CO2/1 -> Vds gas vol/3, P8/2
  P8/1 -> P9/2, P10/1
  P10/1 -> sum2/4, N2O,O2 CO2,N23/3
  N2O,O2 CO2,N23/1 -> Exp flow  Out:/1
  N2O,O2 CO2,N22/1 -> Insp flow  Out:/1
  Exp flow in/1 -> N2O,O2 CO2,N2/1
  Insp flow in/1 -> N2O,O2 CO2,N21/1
  N2O,O2 CO2,N21/1 -> sum/4
  N2O,O2 CO2,N21/3 -> sum2/3
  P4/1 -> N2O,O2 CO2,N22/1, sum/2
  P9/1 -> N2O,O2 CO2,N22/3, sum2/1
  sum3/1 -> N2/1
  P12/1 -> P13/2, P11/2
  N2O,O2 CO2,N21/4 -> sum3/3
  P13/1 -> sum3/1, N2O,O2 CO2,N22/4
  P3/1 -> P7/2, P6/1
  P11/1 -> sum3/4, N2O,O2 CO2,N23/4
  N2/1 -> P12/2, Vds gas vol/4
  N2O,O2 CO2,N21/2 -> sum1/3
  N2O,O2 CO2,N2/1 -> sum/3, mdot_exp/1
  N2O,O2 CO2,N2/2 -> sum1/1, mdot_exp/2
  N2O,O2 CO2,N2/3 -> sum2/2, mdot_exp/3
  N2O,O2 CO2,N2/4 -> sum3/2, mdot_exp/4
  mdot_exp/1 -> P5/2, P6/2, P10/2, P11/1, mdot exp total/1

== system Resp18e_updatedPulse/Patient/Airways + alveoli/Series deadspace medium HiVQ 2 ==
  Insp flow in : Inport  PortDimensions=4  OutDataType=sfix(16)  OutScaling=2^0
  Exp flow in : Inport  Port=2  PortDimensions=4  OutDataType=sfix(16)  OutScaling=2^0
  1/u : Math  Operator=reciprocal  OutDataType=sfix(16)  OutScaling=2^0  SaturateOnIntegerOverflow=on
  CO2 : Integrator  InitialCondition=m_CO2_ds_med_hivq2_i
  N2 : Integrator  InitialCondition=m_N2_ds_med_hivq2_i
  N2O : Integrator  InitialCondition=m_N2O_ds_med_hivq2_i
  N2O O2 CO2 N2 : Demux
  "N2O O2 CO2 N2 " : Demux
  N2O,O2 CO2,N22 : Mux
  N2O,O2 CO2,N23 : Mux
  O2 : Integrator  InitialCondition=m_O2_ds_med_hivq2_i
  P{2..13} (12 alike) : Product  OutDataType=sfix(16)  OutScaling=2^0  SaturateOnIntegerOverflow=on  RndMeth=Zero  InputSameDT=on  OutDataTypeStr=Inherit: Same as first input
  Vds gas vol : Sum  Inputs=++++  OutDataType=sfix(16)  OutScaling=2^0  SaturateOnIntegerOverflow=on  InputSameDT=on  OutDataTypeStr=Inherit: Same as first input
  sum : Sum  Inputs=--++  OutDataType=sfix(16)  OutScaling=2^0  SaturateOnIntegerOverflow=on  InputSameDT=on  OutDataTypeStr=Inherit: Same as first input
  sum1 : Sum  Inputs=+-+-  OutDataType=sfix(16)  OutScaling=2^0  SaturateOnIntegerOverflow=on  InputSameDT=on  OutDataTypeStr=Inherit: Same as first input
  sum2 : Sum  Inputs=-++-  OutDataType=sfix(16)  OutScaling=2^0  SaturateOnIntegerOverflow=on  InputSameDT=on  OutDataTypeStr=Inherit: Same as first input
  sum3 : Sum  Inputs=-++-  OutDataType=sfix(16)  OutScaling=2^0  SaturateOnIntegerOverflow=on  InputSameDT=on  OutDataTypeStr=Inherit: Same as first input
  sum4 : Sum  Inputs=++++  OutDataType=sfix(16)  OutScaling=2^0  SaturateOnIntegerOverflow=on  InputSameDT=on  OutDataTypeStr=Inherit: Same as first input
  sum5 : Sum  Inputs=++++  OutDataType=sfix(16)  OutScaling=2^0  SaturateOnIntegerOverflow=on  InputSameDT=on  OutDataTypeStr=Inherit: Same as first input
  Insp flow  Out: : Outport  OutDataType=sfix(16)  OutScaling=2^0
  Exp flow  Out: : Outport  Port=2  OutDataType=sfix(16)  OutScaling=2^0
  wires:
  P11/1 -> N2O,O2 CO2,N23/4, sum3/4
  P3/1 -> P7/2, P6/1
  P13/1 -> N2O,O2 CO2,N22/4, sum3/1
  P12/1 -> P13/2, P11/2
  sum3/1 -> N2/1
  P9/1 -> sum2/1, N2O,O2 CO2,N22/3
  P4/1 -> sum/2, N2O,O2 CO2,N22/1
  N2O,O2 CO2,N22/1 -> Insp flow  Out:/1
  N2O,O2 CO2,N23/1 -> Exp flow  Out:/1
  P10/1 -> N2O,O2 CO2,N23/3, sum2/4
  P8/1 -> P9/2, P10/1
  CO2/1 -> Vds gas vol/3, P8/2
  P2/1 -> P4/2, P5/1
  sum2/1 -> CO2/1
  sum/1 -> N2O/1
  sum1/1 -> O2/1
  Vds gas vol/1 -> 1/u/1
  1/u/1 -> P12/1, P8/1, P3/1, P2/2
  P7/1 -> N2O,O2 CO2,N22/2, sum1/2
  N2O/1 -> P2/1, Vds gas vol/1
  O2/1 -> P3/2, Vds gas vol/2
  P6/1 -> N2O,O2 CO2,N23/2, sum1/4
  P5/1 -> N2O,O2 CO2,N23/1, sum/1
  N2/1 -> P12/2, Vds gas vol/4
  sum4/1 -> P4/1, P7/1, P9/1, P13/1
  sum5/1 -> P11/1, P10/2, P5/2, P6/2
  N2O O2 CO2 N2/1 -> sum/3, sum5/1
  N2O O2 CO2 N2/2 -> sum1/1, sum5/2
  N2O O2 CO2 N2/3 -> sum2/2, sum5/3
  N2O O2 CO2 N2/4 -> sum3/2, sum5/4
  Exp flow in/1 -> N2O O2 CO2 N2/1
  "N2O O2 CO2 N2 "/1 -> sum/4, sum4/1
  "N2O O2 CO2 N2 "/2 -> sum1/3, sum4/2
  "N2O O2 CO2 N2 "/3 -> sum2/3, sum4/3
  "N2O O2 CO2 N2 "/4 -> sum3/3, sum4/4
  Insp flow in/1 -> "N2O O2 CO2 N2 "/1

== system Resp18e_updatedPulse/Patient/Airways + alveoli/Series deadspace medium hiVQ 1 ==
  Insp flow in : Inport  PortDimensions=4  OutDataType=sfix(16)  OutScaling=2^0
  Exp flow in : Inport  Port=2  PortDimensions=4  OutDataType=sfix(16)  OutScaling=2^0
  1/u : Math  Operator=reciprocal  OutDataType=sfix(16)  OutScaling=2^0  SaturateOnIntegerOverflow=on
  CO2 : Integrator  InitialCondition=m_CO2_ds_med_hivq1_i
  N2 : Integrator  InitialCondition=m_N2_ds_med_hivq1_i
  N2O : Integrator  InitialCondition=m_N2O_ds_med_hivq1_i
  N2O O2 CO2 N2 : Demux
  "N2O O2 CO2 N2 " : Demux
  N2O,O2 CO2,N22 : Mux
  N2O,O2 CO2,N23 : Mux
  O2 : Integrator  InitialCondition=m_O2_ds_med_hivq1_i
  P{2..13} (12 alike) : Product  OutDataType=sfix(16)  OutScaling=2^0  SaturateOnIntegerOverflow=on  RndMeth=Zero  InputSameDT=on  OutDataTypeStr=Inherit: Same as first input
  Vds gas vol : Sum  Inputs=++++  OutDataType=sfix(16)  OutScaling=2^0  SaturateOnIntegerOverflow=on  InputSameDT=on  OutDataTypeStr=Inherit: Same as first input
  sum : Sum  Inputs=--++  OutDataType=sfix(16)  OutScaling=2^0  SaturateOnIntegerOverflow=on  InputSameDT=on  OutDataTypeStr=Inherit: Same as first input
  sum1 : Sum  Inputs=+-+-  OutDataType=sfix(16)  OutScaling=2^0  SaturateOnIntegerOverflow=on  InputSameDT=on  OutDataTypeStr=Inherit: Same as first input
  sum2 : Sum  Inputs=-++-  OutDataType=sfix(16)  OutScaling=2^0  SaturateOnIntegerOverflow=on  InputSameDT=on  OutDataTypeStr=Inherit: Same as first input
  sum3 : Sum  Inputs=-++-  OutDataType=sfix(16)  OutScaling=2^0  SaturateOnIntegerOverflow=on  InputSameDT=on  OutDataTypeStr=Inherit: Same as first input
  sum4 : Sum  Inputs=++++  OutDataType=sfix(16)  OutScaling=2^0  SaturateOnIntegerOverflow=on  InputSameDT=on  OutDataTypeStr=Inherit: Same as first input
  sum5 : Sum  Inputs=++++  OutDataType=sfix(16)  OutScaling=2^0  SaturateOnIntegerOverflow=on  InputSameDT=on  OutDataTypeStr=Inherit: Same as first input
  Insp flow  Out: : Outport  OutDataType=sfix(16)  OutScaling=2^0
  Exp flow  Out: : Outport  Port=2  OutDataType=sfix(16)  OutScaling=2^0
  wires:
  Insp flow in/1 -> "N2O O2 CO2 N2 "/1
  "N2O O2 CO2 N2 "/4 -> sum4/4, sum3/3
  "N2O O2 CO2 N2 "/3 -> sum4/3, sum2/3
  "N2O O2 CO2 N2 "/2 -> sum4/2, sum1/3
  "N2O O2 CO2 N2 "/1 -> sum4/1, sum/4
  Exp flow in/1 -> N2O O2 CO2 N2/1
  N2O O2 CO2 N2/4 -> sum5/4, sum3/2
  N2O O2 CO2 N2/3 -> sum5/3, sum2/2
  N2O O2 CO2 N2/2 -> sum5/2, sum1/1
  N2O O2 CO2 N2/1 -> sum5/1, sum/3
  sum5/1 -> P6/2, P5/2, P10/2, P11/1
  sum4/1 -> P13/1, P9/1, P7/1, P4/1
  N2/1 -> Vds gas vol/4, P12/2
  P5/1 -> sum/1, N2O,O2 CO2,N23/1
  P6/1 -> sum1/4, N2O,O2 CO2,N23/2
  O2/1 -> Vds gas vol/2, P3/2
  N2O/1 -> Vds gas vol/1, P2/1
  P7/1 -> sum1/2, N2O,O2 CO2,N22/2
  1/u/1 -> P2/2, P3/1, P8/1, P12/1
  Vds gas vol/1 -> 1/u/1
  sum1/1 -> O2/1
  sum/1 -> N2O/1
  sum2/1 -> CO2/1
  P2/1 -> P5/1, P4/2
  CO2/1 -> P8/2, Vds gas vol/3
  P8/1 -> P10/1, P9/2
  P10/1 -> sum2/4, N2O,O2 CO2,N23/3
  N2O,O2 CO2,N23/1 -> Exp flow  Out:/1
  N2O,O2 CO2,N22/1 -> Insp flow  Out:/1
  P4/1 -> N2O,O2 CO2,N22/1, sum/2
  P9/1 -> N2O,O2 CO2,N22/3, sum2/1
  sum3/1 -> N2/1
  P12/1 -> P11/2, P13/2
  P13/1 -> sum3/1, N2O,O2 CO2,N22/4
  P3/1 -> P6/1, P7/2
  P11/1 -> sum3/4, N2O,O2 CO2,N23/4

== system Resp18e_updatedPulse/Patient/Airways + alveoli/Series deadspace medium med_lo VQ 1 ==
  Insp flow in : Inport  PortDimensions=4  OutDataType=sfix(16)  OutScaling=2^0
  Exp flow in : Inport  Port=2  PortDimensions=4  OutDataType=sfix(16)  OutScaling=2^0
  1/u : Math  Operator=reciprocal  OutDataType=sfix(16)  OutScaling=2^0  SaturateOnIntegerOverflow=on
  CO2 : Integrator  InitialCondition=m_CO2_ds_med_lovq1_i
  N2 : Integrator  InitialCondition=m_N2_ds_med_lovq1_i
  N2O : Integrator  InitialCondition=m_N2O_ds_med_lovq1_i
  N2O O2 CO2 N2 : Demux
  "N2O O2 CO2 N2 " : Demux
  N2O,O2 CO2,N22 : Mux
  N2O,O2 CO2,N23 : Mux
  O2 : Integrator  InitialCondition=m_O2_ds_med_lovq1_i
  P{2..13} (12 alike) : Product  OutDataType=sfix(16)  OutScaling=2^0  SaturateOnIntegerOverflow=on  RndMeth=Zero  InputSameDT=on  OutDataTypeStr=Inherit: Same as first input
  Vds gas vol : Sum  Inputs=++++  OutDataType=sfix(16)  OutScaling=2^0  SaturateOnIntegerOverflow=on  InputSameDT=on  OutDataTypeStr=Inherit: Same as first input
  sum : Sum  Inputs=--++  OutDataType=sfix(16)  OutScaling=2^0  SaturateOnIntegerOverflow=on  InputSameDT=on  OutDataTypeStr=Inherit: Same as first input
  sum1 : Sum  Inputs=+-+-  OutDataType=sfix(16)  OutScaling=2^0  SaturateOnIntegerOverflow=on  InputSameDT=on  OutDataTypeStr=Inherit: Same as first input
  sum2 : Sum  Inputs=-++-  OutDataType=sfix(16)  OutScaling=2^0  SaturateOnIntegerOverflow=on  InputSameDT=on  OutDataTypeStr=Inherit: Same as first input
  sum3 : Sum  Inputs=-++-  OutDataType=sfix(16)  OutScaling=2^0  SaturateOnIntegerOverflow=on  InputSameDT=on  OutDataTypeStr=Inherit: Same as first input
  sum4 : Sum  Inputs=++++  OutDataType=sfix(16)  OutScaling=2^0  SaturateOnIntegerOverflow=on  InputSameDT=on  OutDataTypeStr=Inherit: Same as first input
  sum5 : Sum  Inputs=++++  OutDataType=sfix(16)  OutScaling=2^0  SaturateOnIntegerOverflow=on  InputSameDT=on  OutDataTypeStr=Inherit: Same as first input
  Insp flow  Out: : Outport  OutDataType=sfix(16)  OutScaling=2^0
  Exp flow  Out: : Outport  Port=2  OutDataType=sfix(16)  OutScaling=2^0
  wires:
  P11/1 -> N2O,O2 CO2,N23/4, sum3/4
  P3/1 -> P7/2, P6/1
  P13/1 -> N2O,O2 CO2,N22/4, sum3/1
  P12/1 -> P13/2, P11/2
  sum3/1 -> N2/1
  P9/1 -> sum2/1, N2O,O2 CO2,N22/3
  P4/1 -> sum/2, N2O,O2 CO2,N22/1
  N2O,O2 CO2,N22/1 -> Insp flow  Out:/1
  N2O,O2 CO2,N23/1 -> Exp flow  Out:/1
  P10/1 -> N2O,O2 CO2,N23/3, sum2/4
  P8/1 -> P9/2, P10/1
  CO2/1 -> Vds gas vol/3, P8/2
  P2/1 -> P4/2, P5/1
  sum2/1 -> CO2/1
  sum/1 -> N2O/1
  sum1/1 -> O2/1
  Vds gas vol/1 -> 1/u/1
  1/u/1 -> P12/1, P8/1, P3/1, P2/2
  P7/1 -> N2O,O2 CO2,N22/2, sum1/2
  N2O/1 -> P2/1, Vds gas vol/1
  O2/1 -> P3/2, Vds gas vol/2
  P6/1 -> N2O,O2 CO2,N23/2, sum1/4
  P5/1 -> N2O,O2 CO2,N23/1, sum/1
  N2/1 -> P12/2, Vds gas vol/4
  sum4/1 -> P4/1, P7/1, P9/1, P13/1
  sum5/1 -> P11/1, P10/2, P5/2, P6/2
  N2O O2 CO2 N2/1 -> sum/3, sum5/1
  N2O O2 CO2 N2/2 -> sum1/1, sum5/2
  N2O O2 CO2 N2/3 -> sum2/2, sum5/3
  N2O O2 CO2 N2/4 -> sum3/2, sum5/4
  Exp flow in/1 -> N2O O2 CO2 N2/1
  "N2O O2 CO2 N2 "/1 -> sum/4, sum4/1
  "N2O O2 CO2 N2 "/2 -> sum1/3, sum4/2
  "N2O O2 CO2 N2 "/3 -> sum2/3, sum4/3
  "N2O O2 CO2 N2 "/4 -> sum3/3, sum4/4
  Insp flow in/1 -> "N2O O2 CO2 N2 "/1

== system Resp18e_updatedPulse/Patient/Airways + alveoli/Series deadspace medium med_loVQ 2 ==
  Insp flow in : Inport  PortDimensions=4  OutDataType=sfix(16)  OutScaling=2^0
  Exp flow in : Inport  Port=2  PortDimensions=4  OutDataType=sfix(16)  OutScaling=2^0
  1/u : Math  Operator=reciprocal  OutDataType=sfix(16)  OutScaling=2^0  SaturateOnIntegerOverflow=on
  CO2 : Integrator  InitialCondition=m_CO2_ds_med_lovq2_i
  N2 : Integrator  InitialCondition=m_N2_ds_med_lovq2_i
  N2O : Integrator  InitialCondition=m_N2O_ds_med_lovq2_i
  N2O O2 CO2 N2 : Demux
  "N2O O2 CO2 N2 " : Demux
  N2O,O2 CO2,N22 : Mux
  N2O,O2 CO2,N23 : Mux
  O2 : Integrator  InitialCondition=m_O2_ds_med_lovq2_i
  P{2..13} (12 alike) : Product  OutDataType=sfix(16)  OutScaling=2^0  SaturateOnIntegerOverflow=on  RndMeth=Zero  InputSameDT=on  OutDataTypeStr=Inherit: Same as first input
  Vds gas vol : Sum  Inputs=++++  OutDataType=sfix(16)  OutScaling=2^0  SaturateOnIntegerOverflow=on  InputSameDT=on  OutDataTypeStr=Inherit: Same as first input
  sum : Sum  Inputs=--++  OutDataType=sfix(16)  OutScaling=2^0  SaturateOnIntegerOverflow=on  InputSameDT=on  OutDataTypeStr=Inherit: Same as first input
  sum1 : Sum  Inputs=+-+-  OutDataType=sfix(16)  OutScaling=2^0  SaturateOnIntegerOverflow=on  InputSameDT=on  OutDataTypeStr=Inherit: Same as first input
  sum2 : Sum  Inputs=-++-  OutDataType=sfix(16)  OutScaling=2^0  SaturateOnIntegerOverflow=on  InputSameDT=on  OutDataTypeStr=Inherit: Same as first input
  sum3 : Sum  Inputs=-++-  OutDataType=sfix(16)  OutScaling=2^0  SaturateOnIntegerOverflow=on  InputSameDT=on  OutDataTypeStr=Inherit: Same as first input
  sum4 : Sum  Inputs=++++  OutDataType=sfix(16)  OutScaling=2^0  SaturateOnIntegerOverflow=on  InputSameDT=on  OutDataTypeStr=Inherit: Same as first input
  sum5 : Sum  Inputs=++++  OutDataType=sfix(16)  OutScaling=2^0  SaturateOnIntegerOverflow=on  InputSameDT=on  OutDataTypeStr=Inherit: Same as first input
  Insp flow  Out: : Outport  OutDataType=sfix(16)  OutScaling=2^0
  Exp flow  Out: : Outport  Port=2  OutDataType=sfix(16)  OutScaling=2^0
  wires:
  Insp flow in/1 -> "N2O O2 CO2 N2 "/1
  "N2O O2 CO2 N2 "/4 -> sum4/4, sum3/3
  "N2O O2 CO2 N2 "/3 -> sum4/3, sum2/3
  "N2O O2 CO2 N2 "/2 -> sum4/2, sum1/3
  "N2O O2 CO2 N2 "/1 -> sum4/1, sum/4
  Exp flow in/1 -> N2O O2 CO2 N2/1
  N2O O2 CO2 N2/4 -> sum5/4, sum3/2
  N2O O2 CO2 N2/3 -> sum5/3, sum2/2
  N2O O2 CO2 N2/2 -> sum5/2, sum1/1
  N2O O2 CO2 N2/1 -> sum5/1, sum/3
  sum5/1 -> P6/2, P5/2, P10/2, P11/1
  sum4/1 -> P13/1, P9/1, P7/1, P4/1
  N2/1 -> Vds gas vol/4, P12/2
  P5/1 -> sum/1, N2O,O2 CO2,N23/1
  P6/1 -> sum1/4, N2O,O2 CO2,N23/2
  O2/1 -> Vds gas vol/2, P3/2
  N2O/1 -> Vds gas vol/1, P2/1
  P7/1 -> sum1/2, N2O,O2 CO2,N22/2
  1/u/1 -> P2/2, P3/1, P8/1, P12/1
  Vds gas vol/1 -> 1/u/1
  sum1/1 -> O2/1
  sum/1 -> N2O/1
  sum2/1 -> CO2/1
  P2/1 -> P5/1, P4/2
  CO2/1 -> P8/2, Vds gas vol/3
  P8/1 -> P10/1, P9/2
  P10/1 -> sum2/4, N2O,O2 CO2,N23/3
  N2O,O2 CO2,N23/1 -> Exp flow  Out:/1
  N2O,O2 CO2,N22/1 -> Insp flow  Out:/1
  P4/1 -> N2O,O2 CO2,N22/1, sum/2
  P9/1 -> N2O,O2 CO2,N22/3, sum2/1
  sum3/1 -> N2/1
  P12/1 -> P11/2, P13/2
  P13/1 -> sum3/1, N2O,O2 CO2,N22/4
  P3/1 -> P6/1, P7/2
  P11/1 -> sum3/4, N2O,O2 CO2,N23/4

== system Resp18e_updatedPulse/Patient/Anaesthetic Machine & resp mechanics/Insp gas mixing ==
  note: Gas mixing subsystem
  note: moles/sec
  note: moles/sec
  note: moles/sec
  note: CO2 can be gated to be inspired only during early part of tidal vol so
      | minimal CO2 is left in the dead space at the end of each inspiration
  mdot_insp : Inport  OutDataType=sfix(16)  OutScaling=2^0
  O_2 : Inport  Port=2  OutDataType=fixdt(1, 16)  OutScaling=2^0
  CO_2 : Inport  Port=3  OutDataType=fixdt(1, 16)  OutScaling=2^0
  N_2 : Inport  Port=4  OutDataType=fixdt(1, 16)  OutScaling=2^0
  Abs : Abs  SaturateOnIntegerOverflow=on
  CO2 : Product  OutDataType=sfix(16)  OutScaling=2^0  SaturateOnIntegerOverflow=on  RndMeth=Zero  InputSameDT=on  OutDataTypeStr=Inherit: Same as first input
  Constant : Constant  OutDataType=sfix(16)  OutScaling=2^0
  Constant1 : Constant  Value=Fi_error  OutDataType=sfix(16)  OutScaling=2^0
  FiN2O : Constant  Value=0  OutDataType=sfix(16)  OutScaling=2^0
  Insp gas calcs : Subsystem
  Mux N2O O2 CO2 N2 : Mux
  N2 : Product  OutDataType=sfix(16)  OutScaling=2^0  SaturateOnIntegerOverflow=on  RndMeth=Zero  InputSameDT=on  OutDataTypeStr=Inherit: Same as first input
  N2O : Product  OutDataType=sfix(16)  OutScaling=2^0  SaturateOnIntegerOverflow=on  RndMeth=Zero  InputSameDT=on  OutDataTypeStr=Inherit: Same as first input
  O2 : Product  OutDataType=sfix(16)  OutScaling=2^0  SaturateOnIntegerOverflow=on  RndMeth=Zero  InputSameDT=on  OutDataTypeStr=Inherit: Same as first input
  Relational Operator : RelationalOperator  Operator=>  InputSameDT=on
  Stop Simulation : Stop
  Sum : Sum  Inputs=++++  OutDataType=sfix(16)  OutScaling=2^0  SaturateOnIntegerOverflow=on  InputSameDT=on  OutDataTypeStr=Inherit: Same as first input
  Tidal vol6 : Sum  Inputs=+-  OutDataType=sfix(16)  OutScaling=2^0  SaturateOnIntegerOverflow=on  InputSameDT=on  OutDataTypeStr=Inherit: Same as first input
  To WS4 : ToWorkspace  VariableName=Fi_CO2  SampleTime=t_sample  SaveFormat=Array
  To WS5 : ToWorkspace  VariableName=Fi_N2  SampleTime=t_sample  SaveFormat=Array
  To WS6 : ToWorkspace  VariableName=Fi_O2  SampleTime=t_sample  SaveFormat=Array
  Insp flow : Outport  OutDataType=sfix(16)  OutScaling=2^0
  wires:
  N2/1 -> Mux N2O O2 CO2 N2/4
  N2O/1 -> Mux N2O O2 CO2 N2/1
  O2/1 -> Mux N2O O2 CO2 N2/2
  CO2/1 -> Mux N2O O2 CO2 N2/3
  mdot_insp/1 -> N2/1, CO2/1, O2/1, N2O/1
  Relational Operator/1 -> Stop Simulation/1
  Abs/1 -> Relational Operator/1
  Constant1/1 -> Relational Operator/2
  Constant/1 -> Tidal vol6/2
  Tidal vol6/1 -> Abs/1
  Sum/1 -> Tidal vol6/1
  FiN2O/1 -> N2O/2, Sum/1
  Mux N2O O2 CO2 N2/1 -> Insp flow/1
  CO_2/1 -> Sum/3, CO2/2, To WS4/1
  N_2/1 -> Sum/4, N2/2, To WS5/1
  O_2/1 -> Sum/2, O2/2, To WS6/1
